simulink model "simmm"  (R2020b)
settings: Solver=VariableStepAuto  StartTime=0.0  StopTime=8  RelTol=1e-4
values from neighbouring files (symbols this model uses):
  b = 0.1    [invertedpendulum.m]
  g = 9.8    [invertedpendulum.m]
  I = 0.006    [invertedpendulum.m]
  Kinf = ((R+(B')*Pinf*B)^-1)*B'*Pinf*A    [invertedpendulum.m]
  l = 0.3    [invertedpendulum.m]
  M = 0.5    [invertedpendulum.m]
  m = 0.2    [invertedpendulum.m]
  T = 1e-1    (= 0.1)    [invertedpendulum.m]
libraries: simulink_extras x5
settings Model: SimulationMode=accelerator  Creator=mehme  LastModifiedBy=mehme
settings SolverCC: AlgebraicLoopSolver=LineSearch

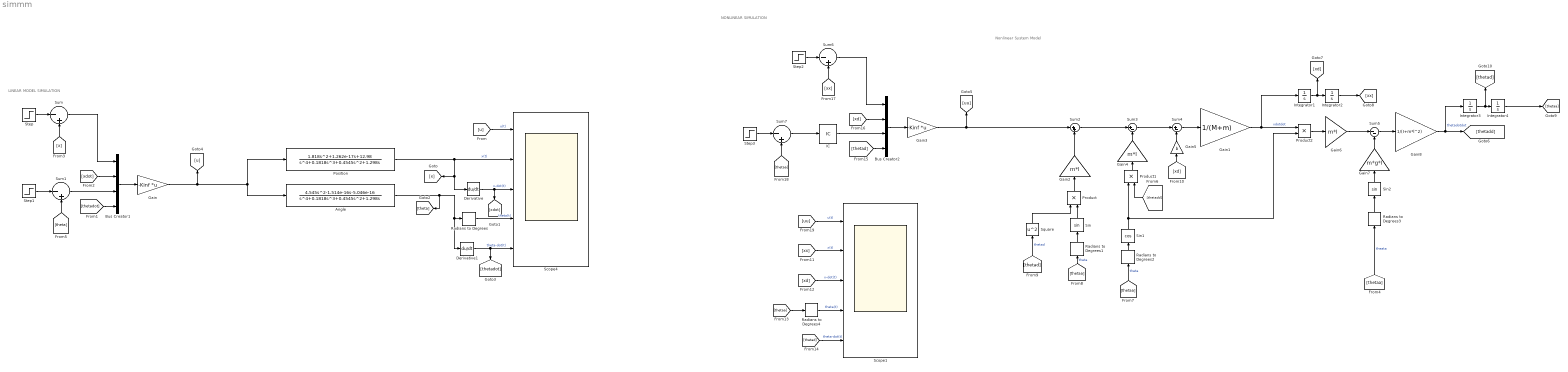
== system simmm ==
  note: NONLINEAR SIMULATION
  note: Nonlinear System Model
  note: LINEAR MODEL SIMULATION
  Angle : TransferFcn  Numerator=[4.545 -1.514e-16 -5.046e-16]  Denominator=[1 0.1818 0.4545 1.298 0]  ContinuousStateAttributes='theta'
  Bus Creator1 : BusCreator  Inputs=4
  Bus Creator2 : BusCreator  Inputs=4
  Derivative : Derivative
  Derivative1 : Derivative
  Gain : Gain  Gain=-Kinf  Multiplication=Matrix(K*u) (u vector)
  Gain1 : Gain  Gain=1/(M+m)
  Gain2 : Gain  Gain=m*l
  Gain3 : Gain  Gain=-Kinf  Multiplication=Matrix(K*u) (u vector)
  Gain4 : Gain  Gain=m*l
  Gain5 : Gain  Gain=b
  Gain6 : Gain  Gain=m*l
  Gain7 : Gain  Gain=m*g*l
  Gain8 : Gain  Gain=1/(I+m*l^2)
  IC : InitialCondition  Value=2
  Integrator{1..4} (4 alike) : Integrator
  Position : TransferFcn  Numerator=[1.818 1.262e-17 12.98]  Denominator=[1 0.1818 0.4545 1.298 0]  ContinuousStateAttributes='x'
  Product : Product
  Product1 : Product
  Product2 : Product
  Radians to Degrees{,1..4} (5 alike) : simulink_extras/Transformations/Radians to Degrees
  Scope1 : Scope  NumInputPorts=5
  Scope4 : Scope  NumInputPorts=5
  Sin : Trigonometry
  Sin1 : Trigonometry  Operator=cos
  Sin2 : Trigonometry
  Square : Math  Operator=square  SaturateOnIntegerOverflow=on
  Step : Step  Time=3  SampleTime=T
  Step1 : Step  Time=3  After=0  SampleTime=T
  Step2 : Step  Time=3  After=0  SampleTime=T
  Step3 : Step  Time=3  After=0  SampleTime=T
  Sum{,1,6..7} (4 alike) : Sum  Inputs=|-+
  Sum2 : Sum  Inputs=|++
  Sum3 : Sum  Inputs=|+-
  Sum4 : Sum  Inputs=|+-
  Sum5 : Sum  Inputs=|--
  wires:
  Derivative1/1 -> Scope4/5, [thetadot]  "theta-dot(t)"
  Sum/1 -> Bus Creator1/1
  Step/1 -> Sum/1
  Bus Creator1/1 -> Gain/1
  [x] -> Sum/2
  [xdot] -> Bus Creator1/2
  [thetadot] -> Bus Creator1/4
  Gain/1 -> [u], Angle/1, Position/1
  Angle/1 -> [theta], Derivative1/1, Radians to Degrees/1
  Position/1 -> Derivative/1, [x], Scope4/2  "x(t)"
  Derivative/1 -> [xdot], Scope4/3  "x-dot(t)"
  [u] -> Scope4/1  "u(t)"
  Radians to Degrees/1 -> Scope4/4  "theta(t)"
  Sum1/1 -> Bus Creator1/3
  [theta] -> Sum1/2
  Step1/1 -> Sum1/1
  Gain3/1 -> Sum2/1, [uu]
  Sum2/1 -> Sum3/1
  Sum3/1 -> Sum4/1
  Sum4/1 -> Gain1/1
  Product/1 -> Gain2/1
  Gain2/1 -> Sum2/2
  Square/1 -> Product/1
  Sin/1 -> Product/2
  Sin1/1 -> Product2/2, Product1/1
  [thetadd] -> Product1/2
  Gain4/1 -> Sum3/2
  Product1/1 -> Gain4/1
  Gain5/1 -> Sum4/2
  [xd] -> Gain5/1
  Gain1/1 -> Product2/1, Integrator1/1  "xdotdot"
  [thetad] -> Square/1  "thetad"
  [thetaa] -> Radians to Degrees1/1  "theta"
  [thetaa] -> Radians to Degrees2/1  "theta"
  Product2/1 -> Gain6/1
  Gain6/1 -> Sum5/1
  [thetaa] -> Radians to Degrees3/1  "theata"
  Sin2/1 -> Gain7/1
  Gain7/1 -> Sum5/2
  Sum5/1 -> Gain8/1
  Gain8/1 -> Integrator3/1, [thetadd]  "thetadotdot"
  Integrator1/1 -> [xd], Integrator2/1
  Integrator3/1 -> [thetad], Integrator4/1
  Integrator2/1 -> [xx]
  [xx] -> Scope1/2  "x(t)"
  [xd] -> Scope1/3  "x-dot(t)"
  [thetad] -> Scope1/5  "theta-dot(t)"
  [thetaa] -> Sum7/2
  Step3/1 -> Sum7/1
  Bus Creator2/1 -> Gain3/1
  Step2/1 -> Sum6/1
  [xd] -> Bus Creator2/2
  Sum6/1 -> Bus Creator2/1
  [xx] -> Sum6/2
  [thetad] -> Bus Creator2/4
  [uu] -> Scope1/1  "u(t)"
  Radians to Degrees1/1 -> Sin/1
  Radians to Degrees2/1 -> Sin1/1
  Radians to Degrees3/1 -> Sin2/1
  [thetaa] -> Radians to Degrees4/1
  Radians to Degrees4/1 -> Scope1/4  "theta(t)"
  Integrator4/1 -> [thetaa]
  Sum7/1 -> IC/1
  IC/1 -> Bus Creator2/3
